simulink model "sf_if"  (Simulink 7.6)
settings: Solver=ode45  StartTime=0.0  StopTime=10.0  MaxStep=.05  RelTol=1e-3
libraries: simulink x1
settings Model: Creator=The MathWorks Inc.  CovMetricSettings=dcmtr  ExtModeAutoUpdateStatusClock=off
settings DataIOCC: SignalLoggingName=sigsOut
settings OptimizationCC: InlineInvariantSignals=on  InitFltsAndDblsToZero=on  EfficientMapNaN2IntZero=off
settings DebuggingCC: SaveWithParameterizedLinksMsg=none  SignalResolutionControl=TryResolveAllWithWarning  SolverPrmCheckMsg=none  MultiTaskDSMMsg=warning  MultiTaskCondExecSysMsg=none  StrictBusMsg=None
settings HardwareCC: TargetUnknown=on
settings SFSimCC: SimParseCustomCode=off
settings RTWCC: IncludeERTFirstTime=on
settings GRTTargetCC: TargetFcnLib=ansi_tfl_tmw.mat

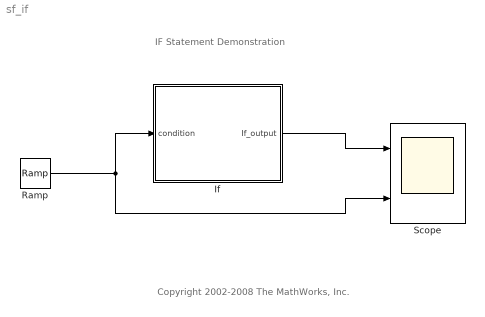
== system sf_if ==
  note: IF Statement Demonstration
  note: Copyright 2002-2008 The MathWorks, Inc.
  If : Stateflow chart  TreatAsAtomicUnit=on
  Ramp : simulink/Sources/Ramp  SystemSampleTime=-1  slope=10  start=0  X0=0
  Scope : Scope  NumInputPorts=2
      settings: TimeRange=10  YMin=-100~0  YMax=400~100
  wires:
  Ramp/1 -> If/1(condition), Scope/2
  If/1(If_output) -> Scope/1

== stateflow chart If ==
  note: Equivalent M-Code:
      |
      | if condition <= 20
      |     If_output = condition^2;
      | elseif condition > 20 & condition <=50
      |    If_output = 50*sin(condition)
      | else
      |    If_ouptut = condition;
      | end
  (default) -> (junction 4)
  (junction 4) -> (junction 5) [order 1] : [condition<=20] {If_output=condition^2;}
  (junction 4) -> (junction 5) [order 3] : {If_output=condition;}
  (junction 4) -> (junction 5) [order 2] : [condition>20 && condition<=70]
      | {If_output=50*sin(condition);}
  (junction 5) -> (junction 6)
  data: condition input double; If_output output double
